simulink model "dspace"  (R2021b)
settings: Solver=FixedStepDiscrete  StartTime=0.0  StopTime=Inf  FixedStep=1e-3  RelTol=1e-3
PostLoadFcn:
  | , if any(exist('dsrtsu_mdlpostloadfcn', 'file') ~= 0), dsrtsu_mdlpostloadfcn('Execute', bdroot); end,
undefined symbols (not defined in the file): ami, amk1_setpoints_1, amk2_setpoints_1, amk3_setpoints_1, amk4_setpoints_1, as, digital, ebs, indicator, mcu_set_dbu_indicator_points, mcu_set_ecu_indicator_points, res_ntm_node_control
libraries: rtican x63, rti1401lib_dio_type3 x4, simulink x4, simulink_extras x1
(part 2 of 16)

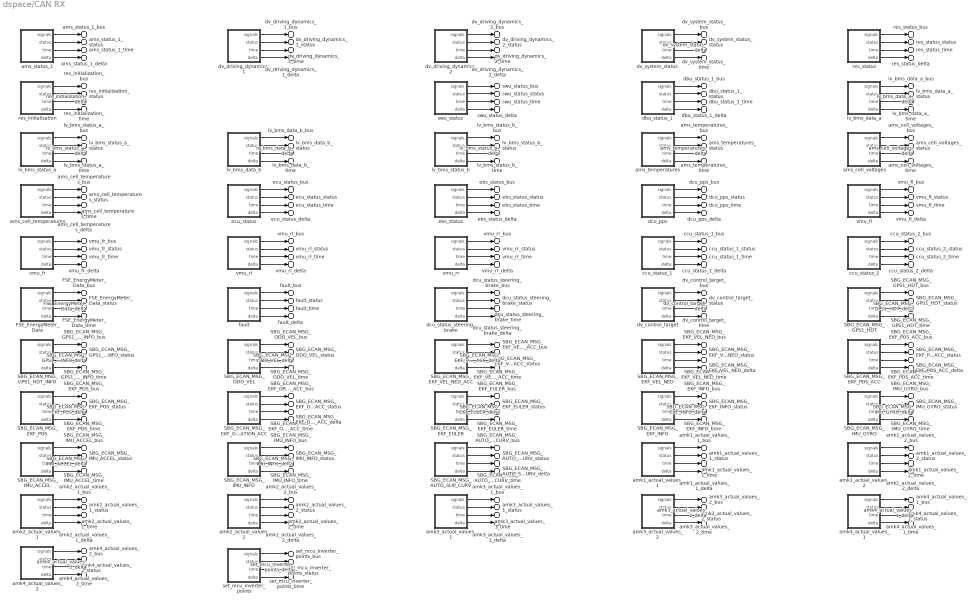
== system dspace/CAN RX ==
  FSE_EnergyMeter_Data : Subsystem
  SBG_ECAN_MSG_AUTO_SLIP_CURV : Subsystem
  SBG_ECAN_MSG_EKF_EULER : Subsystem
  SBG_ECAN_MSG_EKF_INFO : Subsystem
  SBG_ECAN_MSG_EKF_ORIENTATION_ACC : Subsystem
  SBG_ECAN_MSG_EKF_POS : Subsystem
  SBG_ECAN_MSG_EKF_POS_ACC : Subsystem
  SBG_ECAN_MSG_EKF_VEL_NED : Subsystem
  SBG_ECAN_MSG_EKF_VEL_NED_ACC : Subsystem
  SBG_ECAN_MSG_GPS1_HDT : Subsystem
  SBG_ECAN_MSG_GPS1_HDT_INFO : Subsystem
  SBG_ECAN_MSG_IMU_ACCEL : Subsystem
  SBG_ECAN_MSG_IMU_GYRO : Subsystem
  SBG_ECAN_MSG_IMU_INFO : Subsystem
  SBG_ECAN_MSG_ODO_VEL : Subsystem
  amk1_actual_values_1 : Subsystem
  amk1_actual_values_2 : Subsystem
  amk2_actual_values_1 : Subsystem
  amk2_actual_values_2 : Subsystem
  amk3_actual_values_1 : Subsystem
  amk3_actual_values_2 : Subsystem
  amk4_actual_values_1 : Subsystem
  amk4_actual_values_2 : Subsystem
  ams_cell_temperatures : Subsystem
  ams_cell_voltages : Subsystem
  ams_status_1 : Subsystem
  ams_temperatures : Subsystem
  ccu_status_1 : Subsystem
  ccu_status_2 : Subsystem
  dbu_status_1 : Subsystem
  dcu_pps : Subsystem
  dcu_status_steering_brake : Subsystem
  dv_control_target : Subsystem
  dv_driving_dynamics_1 : Subsystem
  dv_driving_dynamics_2 : Subsystem
  dv_system_status : Subsystem
  ebs_status : Subsystem
  ecu_status : Subsystem
  fault : Subsystem
  lv_bms_data_a : Subsystem
  lv_bms_data_b : Subsystem
  lv_bms_status_a : Subsystem
  lv_bms_status_b : Subsystem
  res_initialization : Subsystem
  res_status : Subsystem
  set_mcu_inverter_points : Subsystem
  swu_status : Subsystem
  vmu_fl : Subsystem
  vmu_fr : Subsystem
  vmu_rl : Subsystem
  vmu_rr : Subsystem
  lv_bms_status_a_bus : Outport  PortName=signals  Element=lv_bms_status_a
  lv_bms_data_b_bus : Outport  PortName=signals  Element=lv_bms_data_b
  lv_bms_status_b_bus : Outport  PortName=signals  Element=lv_bms_status_b
  ams_temperatures_bus : Outport  PortName=signals  Element=ams_temperatures
  ams_cell_voltages_bus : Outport  PortName=signals  Element=ams_cell_voltages
  ams_cell_temperatures_bus : Outport  PortName=signals  Element=ams_cell_temperatures
  ecu_status_bus : Outport  PortName=signals  Element=ecu_status
  ebs_status_bus : Outport  PortName=signals  Element=ebs_status
  dcu_pps_bus : Outport  PortName=signals  Element=dcu_pps
  vmu_fl_bus : Outport  PortName=signals  Element=vmu_fl
  vmu_fr_bus : Outport  PortName=signals  Element=vmu_fr
  vmu_rl_bus : Outport  PortName=signals  Element=vmu_rl
  vmu_rr_bus : Outport  PortName=signals  Element=vmu_rr
  ccu_status_1_bus : Outport  PortName=signals  Element=ccu_status_1
  ccu_status_2_bus : Outport  PortName=signals  Element=ccu_status_2
  FSE_EnergyMeter_Data_bus : Outport  PortName=signals  Element=FSE_EnergyMeter_Data
  fault_bus : Outport  PortName=signals  Element=fault
  dcu_status_steering_brake_bus : Outport  PortName=signals  Element=dcu_status_steering_brake
  dv_control_target_bus : Outport  PortName=signals  Element=dv_control_target
  SBG_ECAN_MSG_GPS1_HDT_bus : Outport  PortName=signals  Element=SBG_ECAN_MSG_GPS1_HDT
  SBG_ECAN_MSG_GPS1_HDT_INFO_bus : Outport  PortName=signals  Element=SBG_ECAN_MSG_GPS1_HDT_INFO
  SBG_ECAN_MSG_ODO_VEL_bus : Outport  PortName=signals  Element=SBG_ECAN_MSG_ODO_VEL
  SBG_ECAN_MSG_EKF_VEL_NED_ACC_bus : Outport  PortName=signals  Element=SBG_ECAN_MSG_EKF_VEL_NED_ACC
  SBG_ECAN_MSG_EKF_VEL_NED_bus : Outport  PortName=signals  Element=SBG_ECAN_MSG_EKF_VEL_NED
  SBG_ECAN_MSG_EKF_POS_ACC_bus : Outport  PortName=signals  Element=SBG_ECAN_MSG_EKF_POS_ACC
  SBG_ECAN_MSG_EKF_POS_bus : Outport  PortName=signals  Element=SBG_ECAN_MSG_EKF_POS
  SBG_ECAN_MSG_EKF_ORIENTATION_ACC_bus : Outport  PortName=signals  Element=SBG_ECAN_MSG_EKF_ORIENTATION_ACC
  SBG_ECAN_MSG_EKF_EULER_bus : Outport  PortName=signals  Element=SBG_ECAN_MSG_EKF_EULER
  SBG_ECAN_MSG_EKF_INFO_bus : Outport  PortName=signals  Element=SBG_ECAN_MSG_EKF_INFO
  SBG_ECAN_MSG_IMU_GYRO_bus : Outport  PortName=signals  Element=SBG_ECAN_MSG_IMU_GYRO
  SBG_ECAN_MSG_IMU_ACCEL_bus : Outport  PortName=signals  Element=SBG_ECAN_MSG_IMU_ACCEL
  SBG_ECAN_MSG_IMU_INFO_bus : Outport  PortName=signals  Element=SBG_ECAN_MSG_IMU_INFO
  SBG_ECAN_MSG_AUTO_SLIP_CURV_bus : Outport  PortName=signals  Element=SBG_ECAN_MSG_AUTO_SLIP_CURV
  amk1_actual_values_1_bus : Outport  PortName=signals  Element=amk1_actual_values_1
  amk1_actual_values_2_bus : Outport  PortName=signals  Element=amk1_actual_values_2
  amk2_actual_values_1_bus : Outport  PortName=signals  Element=amk2_actual_values_1
  amk2_actual_values_2_bus : Outport  PortName=signals  Element=amk2_actual_values_2
  amk3_actual_values_1_bus : Outport  PortName=signals  Element=amk3_actual_values_1
  amk3_actual_values_2_bus : Outport  PortName=signals  Element=amk3_actual_values_2
  amk4_actual_values_1_bus : Outport  PortName=signals  Element=amk4_actual_values_1
  amk4_actual_values_2_bus : Outport  PortName=signals  Element=amk4_actual_values_2
  ams_status_1_bus : Outport  PortName=signals  Element=ams_status_1
  dv_driving_dynamics_1_bus : Outport  PortName=signals  Element=dv_driving_dynamics_1
  dv_driving_dynamics_2_bus : Outport  PortName=signals  Element=dv_driving_dynamics_2
  dv_system_status_bus : Outport  PortName=signals  Element=dv_system_status
  res_status_bus : Outport  PortName=signals  Element=res_status
  res_initialization_bus : Outport  PortName=signals  Element=res_initialization
  swu_status_bus : Outport  PortName=signals  Element=swu_status
  dbu_status_1_bus : Outport  PortName=signals  Element=dbu_status_1
  lv_bms_data_a_bus : Outport  PortName=signals  Element=lv_bms_data_a
  set_mcu_inverter_points_bus : Outport  PortName=signals  Element=set_mcu_inverter_points
  lv_bms_status_a_delta : Outport  Port=2  PortName=deltas  Element=lv_bms_status_a_delta
  lv_bms_data_b_delta : Outport  Port=2  PortName=deltas  Element=lv_bms_data_b_delta
  lv_bms_status_b_delta : Outport  Port=2  PortName=deltas  Element=lv_bms_status_b_delta
  ams_temperatures_delta : Outport  Port=2  PortName=deltas  Element=ams_temperatures_delta
  ams_cell_voltages_delta : Outport  Port=2  PortName=deltas  Element=ams_cell_voltages_delta
  ams_cell_temperatures_delta : Outport  Port=2  PortName=deltas  Element=ams_cell_temperatures_delta
  ecu_status_delta : Outport  Port=2  PortName=deltas  Element=ecu_status_delta
  ebs_status_delta : Outport  Port=2  PortName=deltas  Element=ebs_status_delta
  dcu_pps_delta : Outport  Port=2  PortName=deltas  Element=dcu_pps_delta
  vmu_fl_delta : Outport  Port=2  PortName=deltas  Element=vmu_fl_delta
  vmu_fr_delta : Outport  Port=2  PortName=deltas  Element=vmu_fr_delta
  vmu_rl_delta : Outport  Port=2  PortName=deltas  Element=vmu_rl_delta
  vmu_rr_delta : Outport  Port=2  PortName=deltas  Element=vmu_rr_delta
  ccu_status_1_delta : Outport  Port=2  PortName=deltas  Element=ccu_status_1_delta
  ccu_status_2_delta : Outport  Port=2  PortName=deltas  Element=ccu_status_2_delta
  FSE_EnergyMeter_Data_delta : Outport  Port=2  PortName=deltas  Element=FSE_EnergyMeter_Data_delta
  fault_delta : Outport  Port=2  PortName=deltas  Element=fault_delta
  dcu_status_steering_brake_delta : Outport  Port=2  PortName=deltas  Element=dcu_status_steering_brake_delta
  dv_control_target_delta : Outport  Port=2  PortName=deltas  Element=dv_control_target_delta
  SBG_ECAN_MSG_GPS1_HDT_delta : Outport  Port=2  PortName=deltas  Element=SBG_ECAN_MSG_GPS1_HDT_delta
  SBG_ECAN_MSG_GPS1_HDT_INFO_delta : Outport  Port=2  PortName=deltas  Element=SBG_ECAN_MSG_GPS1_HDT_INFO_delta
  SBG_ECAN_MSG_ODO_VEL_delta : Outport  Port=2  PortName=deltas  Element=SBG_ECAN_MSG_ODO_VEL_delta
  SBG_ECAN_MSG_EKF_VEL_NED_ACC_delta : Outport  Port=2  PortName=deltas  Element=SBG_ECAN_MSG_EKF_VEL_NED_ACC_delta
  SBG_ECAN_MSG_EKF_VEL_NED_delta : Outport  Port=2  PortName=deltas  Element=SBG_ECAN_MSG_EKF_VEL_NED_delta
  SBG_ECAN_MSG_EKF_POS_ACC_delta : Outport  Port=2  PortName=deltas  Element=SBG_ECAN_MSG_EKF_POS_ACC_delta
  SBG_ECAN_MSG_EKF_POS_delta : Outport  Port=2  PortName=deltas  Element=SBG_ECAN_MSG_EKF_POS_delta
  SBG_ECAN_MSG_EKF_ORIENTATION_ACC_delta : Outport  Port=2  PortName=deltas  Element=SBG_ECAN_MSG_EKF_ORIENTATION_ACC_delta
  SBG_ECAN_MSG_EKF_EULER_delta : Outport  Port=2  PortName=deltas  Element=SBG_ECAN_MSG_EKF_EULER_delta
  SBG_ECAN_MSG_EKF_INFO_delta : Outport  Port=2  PortName=deltas  Element=SBG_ECAN_MSG_EKF_INFO_delta
  SBG_ECAN_MSG_IMU_GYRO_delta : Outport  Port=2  PortName=deltas  Element=SBG_ECAN_MSG_IMU_GYRO_delta
  SBG_ECAN_MSG_IMU_ACCEL_delta : Outport  Port=2  PortName=deltas  Element=SBG_ECAN_MSG_IMU_ACCEL_delta
  SBG_ECAN_MSG_IMU_INFO_delta : Outport  Port=2  PortName=deltas  Element=SBG_ECAN_MSG_IMU_INFO_delta
  SBG_ECAN_MSG_AUTO_SLIP_CURV_delta : Outport  Port=2  PortName=deltas  Element=SBG_ECAN_MSG_AUTO_SLIP_CURV_delta
  amk1_actual_values_1_delta : Outport  Port=2  PortName=deltas  Element=amk1_actual_values_1_delta
  amk1_actual_values_2_delta : Outport  Port=2  PortName=deltas  Element=amk1_actual_values_2_delta
  amk2_actual_values_1_delta : Outport  Port=2  PortName=deltas  Element=amk2_actual_values_1_delta
  amk2_actual_values_2_delta : Outport  Port=2  PortName=deltas  Element=amk2_actual_values_2_delta
  amk3_actual_values_1_delta : Outport  Port=2  PortName=deltas  Element=amk3_actual_values_1_delta
  amk3_actual_values_2_delta : Outport  Port=2  PortName=deltas  Element=amk3_actual_values_2_delta
  amk4_actual_values_1_delta : Outport  Port=2  PortName=deltas  Element=amk4_actual_values_1_delta
  amk4_actual_values_2_delta : Outport  Port=2  PortName=deltas  Element=amk4_actual_values_2_delta
  ams_status_1_delta : Outport  Port=2  PortName=deltas  Element=ams_status_1_delta
  dv_driving_dynamics_1_delta : Outport  Port=2  PortName=deltas  Element=dv_driving_dynamics_1_delta
  dv_driving_dynamics_2_delta : Outport  Port=2  PortName=deltas  Element=dv_driving_dynamics_2_delta
  dv_system_status_delta : Outport  Port=2  PortName=deltas  Element=dv_system_status_delta
  res_status_delta : Outport  Port=2  PortName=deltas  Element=res_status_delta
  res_initialization_delta : Outport  Port=2  PortName=deltas  Element=res_initialization_delta
  swu_status_delta : Outport  Port=2  PortName=deltas  Element=swu_status_delta
  dbu_status_1_delta : Outport  Port=2  PortName=deltas  Element=dbu_status_1_delta
  lv_bms_data_a_delta : Outport  Port=2  PortName=deltas  Element=lv_bms_data_a_delta
  set_mcu_inverter_points_delta : Outport  Port=2  PortName=deltas  Element=set_mcu_inverter_points_delta
  lv_bms_status_a_status : Outport  Port=3  PortName=status  Element=lv_bms_status_a_status
  lv_bms_data_b_status : Outport  Port=3  PortName=status  Element=lv_bms_data_b_status
  lv_bms_status_b_status : Outport  Port=3  PortName=status  Element=lv_bms_status_b_status
  ams_temperatures_status : Outport  Port=3  PortName=status  Element=ams_temperatures_status
  ams_cell_voltages_status : Outport  Port=3  PortName=status  Element=ams_cell_voltages_status
  ams_cell_temperatures_status : Outport  Port=3  PortName=status  Element=ams_cell_temperatures_status
  ecu_status_status : Outport  Port=3  PortName=status  Element=ecu_status_status
  ebs_status_status : Outport  Port=3  PortName=status  Element=ebs_status_status
  dcu_pps_status : Outport  Port=3  PortName=status  Element=dcu_pps_status
  vmu_fl_status : Outport  Port=3  PortName=status  Element=vmu_fl_status
  vmu_fr_status : Outport  Port=3  PortName=status  Element=vmu_fr_status
  vmu_rl_status : Outport  Port=3  PortName=status  Element=vmu_rl_status
  vmu_rr_status : Outport  Port=3  PortName=status  Element=vmu_rr_status
  ccu_status_1_status : Outport  Port=3  PortName=status  Element=ccu_status_1_status
  ccu_status_2_status : Outport  Port=3  PortName=status  Element=ccu_status_2_status
  FSE_EnergyMeter_Data_status : Outport  Port=3  PortName=status  Element=FSE_EnergyMeter_Data_status
  fault_status : Outport  Port=3  PortName=status  Element=fault_status
  dcu_status_steering_brake_status : Outport  Port=3  PortName=status  Element=dcu_status_steering_brake_status
  dv_control_target_status : Outport  Port=3  PortName=status  Element=dv_control_target_status
  SBG_ECAN_MSG_GPS1_HDT_status : Outport  Port=3  PortName=status  Element=SBG_ECAN_MSG_GPS1_HDT_status
  SBG_ECAN_MSG_GPS1_HDT_INFO_status : Outport  Port=3  PortName=status  Element=SBG_ECAN_MSG_GPS1_HDT_INFO_status
  SBG_ECAN_MSG_ODO_VEL_status : Outport  Port=3  PortName=status  Element=SBG_ECAN_MSG_ODO_VEL_status
  SBG_ECAN_MSG_EKF_VEL_NED_ACC_status : Outport  Port=3  PortName=status  Element=SBG_ECAN_MSG_EKF_VEL_NED_ACC_status
  SBG_ECAN_MSG_EKF_VEL_NED_status : Outport  Port=3  PortName=status  Element=SBG_ECAN_MSG_EKF_VEL_NED_status
  SBG_ECAN_MSG_EKF_POS_ACC_status : Outport  Port=3  PortName=status  Element=SBG_ECAN_MSG_EKF_POS_ACC_status
  SBG_ECAN_MSG_EKF_POS_status : Outport  Port=3  PortName=status  Element=SBG_ECAN_MSG_EKF_POS_status
  SBG_ECAN_MSG_EKF_ORIENTATION_ACC_status : Outport  Port=3  PortName=status  Element=SBG_ECAN_MSG_EKF_ORIENTATION_ACC_status
  SBG_ECAN_MSG_EKF_EULER_status : Outport  Port=3  PortName=status  Element=SBG_ECAN_MSG_EKF_EULER_status
  SBG_ECAN_MSG_EKF_INFO_status : Outport  Port=3  PortName=status  Element=SBG_ECAN_MSG_EKF_INFO_status
  SBG_ECAN_MSG_IMU_GYRO_status : Outport  Port=3  PortName=status  Element=SBG_ECAN_MSG_IMU_GYRO_status
  SBG_ECAN_MSG_IMU_ACCEL_status : Outport  Port=3  PortName=status  Element=SBG_ECAN_MSG_IMU_ACCEL_status
  SBG_ECAN_MSG_IMU_INFO_status : Outport  Port=3  PortName=status  Element=SBG_ECAN_MSG_IMU_INFO_status
  SBG_ECAN_MSG_AUTO_SLIP_CURV_status : Outport  Port=3  PortName=status  Element=SBG_ECAN_MSG_AUTO_SLIP_CURV_status
  amk1_actual_values_1_status : Outport  Port=3  PortName=status  Element=amk1_actual_values_1_status
  amk1_actual_values_2_status : Outport  Port=3  PortName=status  Element=amk1_actual_values_2_status
  amk2_actual_values_1_status : Outport  Port=3  PortName=status  Element=amk2_actual_values_1_status
  amk2_actual_values_2_status : Outport  Port=3  PortName=status  Element=amk2_actual_values_2_status
  amk3_actual_values_1_status : Outport  Port=3  PortName=status  Element=amk3_actual_values_1_status
  amk3_actual_values_2_status : Outport  Port=3  PortName=status  Element=amk3_actual_values_2_status
  amk4_actual_values_1_status : Outport  Port=3  PortName=status  Element=amk4_actual_values_1_status
  amk4_actual_values_2_status : Outport  Port=3  PortName=status  Element=amk4_actual_values_2_status
  ams_status_1_status : Outport  Port=3  PortName=status  Element=ams_status_1_status
  dv_driving_dynamics_1_status : Outport  Port=3  PortName=status  Element=dv_driving_dynamics_1_status
  dv_driving_dynamics_2_status : Outport  Port=3  PortName=status  Element=dv_driving_dynamics_2_status
  dv_system_status_status : Outport  Port=3  PortName=status  Element=dv_system_status_status
  res_status_status : Outport  Port=3  PortName=status  Element=res_status_status
  res_initialization_status : Outport  Port=3  PortName=status  Element=res_initialization_status
  swu_status_status : Outport  Port=3  PortName=status  Element=swu_status_status
  dbu_status_1_status : Outport  Port=3  PortName=status  Element=dbu_status_1_status
  lv_bms_data_a_status : Outport  Port=3  PortName=status  Element=lv_bms_data_a_status
  set_mcu_inverter_points_status : Outport  Port=3  PortName=status  Element=set_mcu_inverter_points_status
  lv_bms_status_a_time : Outport  Port=4  PortName=time  Element=lv_bms_status_a_time
  lv_bms_data_b_time : Outport  Port=4  PortName=time  Element=lv_bms_data_b_time
  lv_bms_status_b_time : Outport  Port=4  PortName=time  Element=lv_bms_status_b_time
  ams_temperatures_time : Outport  Port=4  PortName=time  Element=ams_temperatures_time
  ams_cell_voltages_time : Outport  Port=4  PortName=time  Element=ams_cell_voltages_time
  ams_cell_temperatures_time : Outport  Port=4  PortName=time  Element=ams_cell_temperatures_time
  ecu_status_time : Outport  Port=4  PortName=time  Element=ecu_status_time
  ebs_status_time : Outport  Port=4  PortName=time  Element=ebs_status_time
  dcu_pps_time : Outport  Port=4  PortName=time  Element=dcu_pps_time
  vmu_fl_time : Outport  Port=4  PortName=time  Element=vmu_fl_time
  vmu_fr_time : Outport  Port=4  PortName=time  Element=vmu_fr_time
  vmu_rl_time : Outport  Port=4  PortName=time  Element=vmu_rl_time
  vmu_rr_time : Outport  Port=4  PortName=time  Element=vmu_rr_time
  ccu_status_1_time : Outport  Port=4  PortName=time  Element=ccu_status_1_time
  ccu_status_2_time : Outport  Port=4  PortName=time  Element=ccu_status_2_time
  FSE_EnergyMeter_Data_time : Outport  Port=4  PortName=time  Element=FSE_EnergyMeter_Data_time
  fault_time : Outport  Port=4  PortName=time  Element=fault_time
  dcu_status_steering_brake_time : Outport  Port=4  PortName=time  Element=dcu_status_steering_brake_time
  dv_control_target_time : Outport  Port=4  PortName=time  Element=dv_control_target_time
  SBG_ECAN_MSG_GPS1_HDT_time : Outport  Port=4  PortName=time  Element=SBG_ECAN_MSG_GPS1_HDT_time
  SBG_ECAN_MSG_GPS1_HDT_INFO_time : Outport  Port=4  PortName=time  Element=SBG_ECAN_MSG_GPS1_HDT_INFO_time
  SBG_ECAN_MSG_ODO_VEL_time : Outport  Port=4  PortName=time  Element=SBG_ECAN_MSG_ODO_VEL_time
  SBG_ECAN_MSG_EKF_VEL_NED_ACC_time : Outport  Port=4  PortName=time  Element=SBG_ECAN_MSG_EKF_VEL_NED_ACC_time
  SBG_ECAN_MSG_EKF_VEL_NED_time : Outport  Port=4  PortName=time  Element=SBG_ECAN_MSG_EKF_VEL_NED_time
  SBG_ECAN_MSG_EKF_POS_ACC_time : Outport  Port=4  PortName=time  Element=SBG_ECAN_MSG_EKF_POS_ACC_time
  SBG_ECAN_MSG_EKF_POS_time : Outport  Port=4  PortName=time  Element=SBG_ECAN_MSG_EKF_POS_time
  SBG_ECAN_MSG_EKF_ORIENTATION_ACC_time : Outport  Port=4  PortName=time  Element=SBG_ECAN_MSG_EKF_ORIENTATION_ACC_time
  SBG_ECAN_MSG_EKF_EULER_time : Outport  Port=4  PortName=time  Element=SBG_ECAN_MSG_EKF_EULER_time
  SBG_ECAN_MSG_EKF_INFO_time : Outport  Port=4  PortName=time  Element=SBG_ECAN_MSG_EKF_INFO_time
  SBG_ECAN_MSG_IMU_GYRO_time : Outport  Port=4  PortName=time  Element=SBG_ECAN_MSG_IMU_GYRO_time
  SBG_ECAN_MSG_IMU_ACCEL_time : Outport  Port=4  PortName=time  Element=SBG_ECAN_MSG_IMU_ACCEL_time
  SBG_ECAN_MSG_IMU_INFO_time : Outport  Port=4  PortName=time  Element=SBG_ECAN_MSG_IMU_INFO_time
  SBG_ECAN_MSG_AUTO_SLIP_CURV_time : Outport  Port=4  PortName=time  Element=SBG_ECAN_MSG_AUTO_SLIP_CURV_time
  amk1_actual_values_1_time : Outport  Port=4  PortName=time  Element=amk1_actual_values_1_time
  amk1_actual_values_2_time : Outport  Port=4  PortName=time  Element=amk1_actual_values_2_time
  amk2_actual_values_1_time : Outport  Port=4  PortName=time  Element=amk2_actual_values_1_time
  amk2_actual_values_2_time : Outport  Port=4  PortName=time  Element=amk2_actual_values_2_time
  amk3_actual_values_1_time : Outport  Port=4  PortName=time  Element=amk3_actual_values_1_time
  amk3_actual_values_2_time : Outport  Port=4  PortName=time  Element=amk3_actual_values_2_time
  amk4_actual_values_1_time : Outport  Port=4  PortName=time  Element=amk4_actual_values_1_time
  amk4_actual_values_2_time : Outport  Port=4  PortName=time  Element=amk4_actual_values_2_time
  ams_status_1_time : Outport  Port=4  PortName=time  Element=ams_status_1_time
  dv_driving_dynamics_1_time : Outport  Port=4  PortName=time  Element=dv_driving_dynamics_1_time
  dv_driving_dynamics_2_time : Outport  Port=4  PortName=time  Element=dv_driving_dynamics_2_time
  dv_system_status_time : Outport  Port=4  PortName=time  Element=dv_system_status_time
  res_status_time : Outport  Port=4  PortName=time  Element=res_status_time
  res_initialization_time : Outport  Port=4  PortName=time  Element=res_initialization_time
  swu_status_time : Outport  Port=4  PortName=time  Element=swu_status_time
  dbu_status_1_time : Outport  Port=4  PortName=time  Element=dbu_status_1_time
  lv_bms_data_a_time : Outport  Port=4  PortName=time  Element=lv_bms_data_a_time
  set_mcu_inverter_points_time : Outport  Port=4  PortName=time  Element=set_mcu_inverter_points_time
  wires:
  lv_bms_status_a/1(signals) -> lv_bms_status_a_bus/1
  lv_bms_status_a/2(status) -> lv_bms_status_a_status/1
  lv_bms_status_a/3(time) -> lv_bms_status_a_time/1
  lv_bms_status_a/4(delta) -> lv_bms_status_a_delta/1
  lv_bms_data_b/1(signals) -> lv_bms_data_b_bus/1
  lv_bms_data_b/2(status) -> lv_bms_data_b_status/1
  lv_bms_data_b/3(time) -> lv_bms_data_b_time/1
  lv_bms_data_b/4(delta) -> lv_bms_data_b_delta/1
  lv_bms_status_b/1(signals) -> lv_bms_status_b_bus/1
  lv_bms_status_b/2(status) -> lv_bms_status_b_status/1
  lv_bms_status_b/3(time) -> lv_bms_status_b_time/1
  lv_bms_status_b/4(delta) -> lv_bms_status_b_delta/1
  ams_temperatures/1(signals) -> ams_temperatures_bus/1
  ams_temperatures/2(status) -> ams_temperatures_status/1
  ams_temperatures/3(time) -> ams_temperatures_time/1
  ams_temperatures/4(delta) -> ams_temperatures_delta/1
  ams_cell_voltages/1(signals) -> ams_cell_voltages_bus/1
  ams_cell_voltages/2(status) -> ams_cell_voltages_status/1
  ams_cell_voltages/3(time) -> ams_cell_voltages_time/1
  ams_cell_voltages/4(delta) -> ams_cell_voltages_delta/1
  ams_cell_temperatures/1(signals) -> ams_cell_temperatures_bus/1
  ams_cell_temperatures/2(status) -> ams_cell_temperatures_status/1
  ams_cell_temperatures/3(time) -> ams_cell_temperatures_time/1
  ams_cell_temperatures/4(delta) -> ams_cell_temperatures_delta/1
  ecu_status/1(signals) -> ecu_status_bus/1
  ecu_status/2(status) -> ecu_status_status/1
  ecu_status/3(time) -> ecu_status_time/1
  ecu_status/4(delta) -> ecu_status_delta/1
  ebs_status/1(signals) -> ebs_status_bus/1
  ebs_status/2(status) -> ebs_status_status/1
  ebs_status/3(time) -> ebs_status_time/1
  ebs_status/4(delta) -> ebs_status_delta/1
  dcu_pps/1(signals) -> dcu_pps_bus/1
  dcu_pps/2(status) -> dcu_pps_status/1
  dcu_pps/3(time) -> dcu_pps_time/1
  dcu_pps/4(delta) -> dcu_pps_delta/1
  vmu_fl/1(signals) -> vmu_fl_bus/1
  vmu_fl/2(status) -> vmu_fl_status/1
  vmu_fl/3(time) -> vmu_fl_time/1
  vmu_fl/4(delta) -> vmu_fl_delta/1
  vmu_fr/1(signals) -> vmu_fr_bus/1
  vmu_fr/2(status) -> vmu_fr_status/1
  vmu_fr/3(time) -> vmu_fr_time/1
  vmu_fr/4(delta) -> vmu_fr_delta/1
  vmu_rl/1(signals) -> vmu_rl_bus/1
  vmu_rl/2(status) -> vmu_rl_status/1
  vmu_rl/3(time) -> vmu_rl_time/1
  vmu_rl/4(delta) -> vmu_rl_delta/1
  vmu_rr/1(signals) -> vmu_rr_bus/1
  vmu_rr/2(status) -> vmu_rr_status/1
  vmu_rr/3(time) -> vmu_rr_time/1
  vmu_rr/4(delta) -> vmu_rr_delta/1
  ccu_status_1/1(signals) -> ccu_status_1_bus/1
  ccu_status_1/2(status) -> ccu_status_1_status/1
  ccu_status_1/3(time) -> ccu_status_1_time/1
  ccu_status_1/4(delta) -> ccu_status_1_delta/1
  ccu_status_2/1(signals) -> ccu_status_2_bus/1
  ccu_status_2/2(status) -> ccu_status_2_status/1
  ccu_status_2/3(time) -> ccu_status_2_time/1
  ccu_status_2/4(delta) -> ccu_status_2_delta/1
  FSE_EnergyMeter_Data/1(signals) -> FSE_EnergyMeter_Data_bus/1
  FSE_EnergyMeter_Data/2(status) -> FSE_EnergyMeter_Data_status/1
  FSE_EnergyMeter_Data/3(time) -> FSE_EnergyMeter_Data_time/1
  FSE_EnergyMeter_Data/4(delta) -> FSE_EnergyMeter_Data_delta/1
  fault/1(signals) -> fault_bus/1
  fault/2(status) -> fault_status/1
  fault/3(time) -> fault_time/1
  fault/4(delta) -> fault_delta/1
  dcu_status_steering_brake/1(signals) -> dcu_status_steering_brake_bus/1
  dcu_status_steering_brake/2(status) -> dcu_status_steering_brake_status/1
  dcu_status_steering_brake/3(time) -> dcu_status_steering_brake_time/1
  dcu_status_steering_brake/4(delta) -> dcu_status_steering_brake_delta/1
  dv_control_target/1(signals) -> dv_control_target_bus/1
  dv_control_target/2(status) -> dv_control_target_status/1
  dv_control_target/3(time) -> dv_control_target_time/1
  dv_control_target/4(delta) -> dv_control_target_delta/1
  SBG_ECAN_MSG_GPS1_HDT/1(signals) -> SBG_ECAN_MSG_GPS1_HDT_bus/1
  SBG_ECAN_MSG_GPS1_HDT/2(status) -> SBG_ECAN_MSG_GPS1_HDT_status/1
  SBG_ECAN_MSG_GPS1_HDT/3(time) -> SBG_ECAN_MSG_GPS1_HDT_time/1
  SBG_ECAN_MSG_GPS1_HDT/4(delta) -> SBG_ECAN_MSG_GPS1_HDT_delta/1
  SBG_ECAN_MSG_GPS1_HDT_INFO/1(signals) -> SBG_ECAN_MSG_GPS1_HDT_INFO_bus/1
  SBG_ECAN_MSG_GPS1_HDT_INFO/2(status) -> SBG_ECAN_MSG_GPS1_HDT_INFO_status/1
  SBG_ECAN_MSG_GPS1_HDT_INFO/3(time) -> SBG_ECAN_MSG_GPS1_HDT_INFO_time/1
  SBG_ECAN_MSG_GPS1_HDT_INFO/4(delta) -> SBG_ECAN_MSG_GPS1_HDT_INFO_delta/1
  SBG_ECAN_MSG_ODO_VEL/1(signals) -> SBG_ECAN_MSG_ODO_VEL_bus/1
  SBG_ECAN_MSG_ODO_VEL/2(status) -> SBG_ECAN_MSG_ODO_VEL_status/1
  SBG_ECAN_MSG_ODO_VEL/3(time) -> SBG_ECAN_MSG_ODO_VEL_time/1
  SBG_ECAN_MSG_ODO_VEL/4(delta) -> SBG_ECAN_MSG_ODO_VEL_delta/1
  SBG_ECAN_MSG_EKF_VEL_NED_ACC/1(signals) -> SBG_ECAN_MSG_EKF_VEL_NED_ACC_bus/1
  SBG_ECAN_MSG_EKF_VEL_NED_ACC/2(status) -> SBG_ECAN_MSG_EKF_VEL_NED_ACC_status/1
  SBG_ECAN_MSG_EKF_VEL_NED_ACC/3(time) -> SBG_ECAN_MSG_EKF_VEL_NED_ACC_time/1
  SBG_ECAN_MSG_EKF_VEL_NED_ACC/4(delta) -> SBG_ECAN_MSG_EKF_VEL_NED_ACC_delta/1
  SBG_ECAN_MSG_EKF_VEL_NED/1(signals) -> SBG_ECAN_MSG_EKF_VEL_NED_bus/1
  SBG_ECAN_MSG_EKF_VEL_NED/2(status) -> SBG_ECAN_MSG_EKF_VEL_NED_status/1
  SBG_ECAN_MSG_EKF_VEL_NED/3(time) -> SBG_ECAN_MSG_EKF_VEL_NED_time/1
  SBG_ECAN_MSG_EKF_VEL_NED/4(delta) -> SBG_ECAN_MSG_EKF_VEL_NED_delta/1
  SBG_ECAN_MSG_EKF_POS_ACC/1(signals) -> SBG_ECAN_MSG_EKF_POS_ACC_bus/1
  SBG_ECAN_MSG_EKF_POS_ACC/2(status) -> SBG_ECAN_MSG_EKF_POS_ACC_status/1
  SBG_ECAN_MSG_EKF_POS_ACC/3(time) -> SBG_ECAN_MSG_EKF_POS_ACC_time/1
  SBG_ECAN_MSG_EKF_POS_ACC/4(delta) -> SBG_ECAN_MSG_EKF_POS_ACC_delta/1
  SBG_ECAN_MSG_EKF_POS/1(signals) -> SBG_ECAN_MSG_EKF_POS_bus/1
  SBG_ECAN_MSG_EKF_POS/2(status) -> SBG_ECAN_MSG_EKF_POS_status/1
  SBG_ECAN_MSG_EKF_POS/3(time) -> SBG_ECAN_MSG_EKF_POS_time/1
  SBG_ECAN_MSG_EKF_POS/4(delta) -> SBG_ECAN_MSG_EKF_POS_delta/1
  SBG_ECAN_MSG_EKF_ORIENTATION_ACC/1(signals) -> SBG_ECAN_MSG_EKF_ORIENTATION_ACC_bus/1
  SBG_ECAN_MSG_EKF_ORIENTATION_ACC/2(status) -> SBG_ECAN_MSG_EKF_ORIENTATION_ACC_status/1
  SBG_ECAN_MSG_EKF_ORIENTATION_ACC/3(time) -> SBG_ECAN_MSG_EKF_ORIENTATION_ACC_time/1
  SBG_ECAN_MSG_EKF_ORIENTATION_ACC/4(delta) -> SBG_ECAN_MSG_EKF_ORIENTATION_ACC_delta/1
  SBG_ECAN_MSG_EKF_EULER/1(signals) -> SBG_ECAN_MSG_EKF_EULER_bus/1
  SBG_ECAN_MSG_EKF_EULER/2(status) -> SBG_ECAN_MSG_EKF_EULER_status/1
  SBG_ECAN_MSG_EKF_EULER/3(time) -> SBG_ECAN_MSG_EKF_EULER_time/1
  SBG_ECAN_MSG_EKF_EULER/4(delta) -> SBG_ECAN_MSG_EKF_EULER_delta/1
  SBG_ECAN_MSG_EKF_INFO/1(signals) -> SBG_ECAN_MSG_EKF_INFO_bus/1
  SBG_ECAN_MSG_EKF_INFO/2(status) -> SBG_ECAN_MSG_EKF_INFO_status/1
  SBG_ECAN_MSG_EKF_INFO/3(time) -> SBG_ECAN_MSG_EKF_INFO_time/1
  SBG_ECAN_MSG_EKF_INFO/4(delta) -> SBG_ECAN_MSG_EKF_INFO_delta/1
  SBG_ECAN_MSG_IMU_GYRO/1(signals) -> SBG_ECAN_MSG_IMU_GYRO_bus/1
  SBG_ECAN_MSG_IMU_GYRO/2(status) -> SBG_ECAN_MSG_IMU_GYRO_status/1
  SBG_ECAN_MSG_IMU_GYRO/3(time) -> SBG_ECAN_MSG_IMU_GYRO_time/1
  SBG_ECAN_MSG_IMU_GYRO/4(delta) -> SBG_ECAN_MSG_IMU_GYRO_delta/1
  SBG_ECAN_MSG_IMU_ACCEL/1(signals) -> SBG_ECAN_MSG_IMU_ACCEL_bus/1
  SBG_ECAN_MSG_IMU_ACCEL/2(status) -> SBG_ECAN_MSG_IMU_ACCEL_status/1
  SBG_ECAN_MSG_IMU_ACCEL/3(time) -> SBG_ECAN_MSG_IMU_ACCEL_time/1
  SBG_ECAN_MSG_IMU_ACCEL/4(delta) -> SBG_ECAN_MSG_IMU_ACCEL_delta/1
  SBG_ECAN_MSG_IMU_INFO/1(signals) -> SBG_ECAN_MSG_IMU_INFO_bus/1
  SBG_ECAN_MSG_IMU_INFO/2(status) -> SBG_ECAN_MSG_IMU_INFO_status/1
  SBG_ECAN_MSG_IMU_INFO/3(time) -> SBG_ECAN_MSG_IMU_INFO_time/1
  SBG_ECAN_MSG_IMU_INFO/4(delta) -> SBG_ECAN_MSG_IMU_INFO_delta/1
  SBG_ECAN_MSG_AUTO_SLIP_CURV/1(signals) -> SBG_ECAN_MSG_AUTO_SLIP_CURV_bus/1
  SBG_ECAN_MSG_AUTO_SLIP_CURV/2(status) -> SBG_ECAN_MSG_AUTO_SLIP_CURV_status/1
  SBG_ECAN_MSG_AUTO_SLIP_CURV/3(time) -> SBG_ECAN_MSG_AUTO_SLIP_CURV_time/1
  SBG_ECAN_MSG_AUTO_SLIP_CURV/4(delta) -> SBG_ECAN_MSG_AUTO_SLIP_CURV_delta/1
  amk1_actual_values_1/1(signals) -> amk1_actual_values_1_bus/1
  amk1_actual_values_1/2(status) -> amk1_actual_values_1_status/1
  amk1_actual_values_1/3(time) -> amk1_actual_values_1_time/1
  amk1_actual_values_1/4(delta) -> amk1_actual_values_1_delta/1
  amk1_actual_values_2/1(signals) -> amk1_actual_values_2_bus/1
  amk1_actual_values_2/2(status) -> amk1_actual_values_2_status/1
  amk1_actual_values_2/3(time) -> amk1_actual_values_2_time/1
  amk1_actual_values_2/4(delta) -> amk1_actual_values_2_delta/1
  amk2_actual_values_1/1(signals) -> amk2_actual_values_1_bus/1
  amk2_actual_values_1/2(status) -> amk2_actual_values_1_status/1
  amk2_actual_values_1/3(time) -> amk2_actual_values_1_time/1
  amk2_actual_values_1/4(delta) -> amk2_actual_values_1_delta/1
  amk2_actual_values_2/1(signals) -> amk2_actual_values_2_bus/1
  amk2_actual_values_2/2(status) -> amk2_actual_values_2_status/1
  amk2_actual_values_2/3(time) -> amk2_actual_values_2_time/1
  amk2_actual_values_2/4(delta) -> amk2_actual_values_2_delta/1
  amk3_actual_values_1/1(signals) -> amk3_actual_values_1_bus/1
  amk3_actual_values_1/2(status) -> amk3_actual_values_1_status/1
  amk3_actual_values_1/3(time) -> amk3_actual_values_1_time/1
  amk3_actual_values_1/4(delta) -> amk3_actual_values_1_delta/1
  amk3_actual_values_2/1(signals) -> amk3_actual_values_2_bus/1
  amk3_actual_values_2/2(status) -> amk3_actual_values_2_status/1
  amk3_actual_values_2/3(time) -> amk3_actual_values_2_time/1
  amk3_actual_values_2/4(delta) -> amk3_actual_values_2_delta/1
  amk4_actual_values_1/1(signals) -> amk4_actual_values_1_bus/1
  amk4_actual_values_1/2(status) -> amk4_actual_values_1_status/1
  amk4_actual_values_1/3(time) -> amk4_actual_values_1_time/1
  amk4_actual_values_1/4(delta) -> amk4_actual_values_1_delta/1
  amk4_actual_values_2/1(signals) -> amk4_actual_values_2_bus/1
  amk4_actual_values_2/2(status) -> amk4_actual_values_2_status/1
  amk4_actual_values_2/3(time) -> amk4_actual_values_2_time/1
  amk4_actual_values_2/4(delta) -> amk4_actual_values_2_delta/1
  swu_status/4(delta) -> swu_status_delta/1
  dv_system_status/3(time) -> dv_system_status_time/1
  ams_status_1/3(time) -> ams_status_1_time/1
  dv_driving_dynamics_2/2(status) -> dv_driving_dynamics_2_status/1
  dv_system_status/1(signals) -> dv_system_status_bus/1
  dbu_status_1/1(signals) -> dbu_status_1_bus/1
  dv_driving_dynamics_1/3(time) -> dv_driving_dynamics_1_time/1
  res_initialization/3(time) -> res_initialization_time/1
  dbu_status_1/2(status) -> dbu_status_1_status/1
  res_status/1(signals) -> res_status_bus/1
  swu_status/2(status) -> swu_status_status/1
  lv_bms_data_a/4(delta) -> lv_bms_data_a_delta/1
  res_initialization/4(delta) -> res_initialization_delta/1
  swu_status/3(time) -> swu_status_time/1
  swu_status/1(signals) -> swu_status_bus/1
  res_status/3(time) -> res_status_time/1
  ams_status_1/1(signals) -> ams_status_1_bus/1
  dbu_status_1/3(time) -> dbu_status_1_time/1
  res_status/4(delta) -> res_status_delta/1
  res_initialization/1(signals) -> res_initialization_bus/1
  lv_bms_data_a/3(time) -> lv_bms_data_a_time/1
  dv_driving_dynamics_1/1(signals) -> dv_driving_dynamics_1_bus/1
  res_status/2(status) -> res_status_status/1
  dv_system_status/4(delta) -> dv_system_status_delta/1
  dv_system_status/2(status) -> dv_system_status_status/1
  ams_status_1/2(status) -> ams_status_1_status/1
  dv_driving_dynamics_2/3(time) -> dv_driving_dynamics_2_time/1
  dbu_status_1/4(delta) -> dbu_status_1_delta/1
  res_initialization/2(status) -> res_initialization_status/1
  dv_driving_dynamics_2/1(signals) -> dv_driving_dynamics_2_bus/1
  dv_driving_dynamics_2/4(delta) -> dv_driving_dynamics_2_delta/1
  lv_bms_data_a/2(status) -> lv_bms_data_a_status/1
  dv_driving_dynamics_1/2(status) -> dv_driving_dynamics_1_status/1
  ams_status_1/4(delta) -> ams_status_1_delta/1
  dv_driving_dynamics_1/4(delta) -> dv_driving_dynamics_1_delta/1
  lv_bms_data_a/1(signals) -> lv_bms_data_a_bus/1
  set_mcu_inverter_points/3(time) -> set_mcu_inverter_points_time/1
  set_mcu_inverter_points/1(signals) -> set_mcu_inverter_points_bus/1
  set_mcu_inverter_points/4(delta) -> set_mcu_inverter_points_delta/1
  set_mcu_inverter_points/2(status) -> set_mcu_inverter_points_status/1

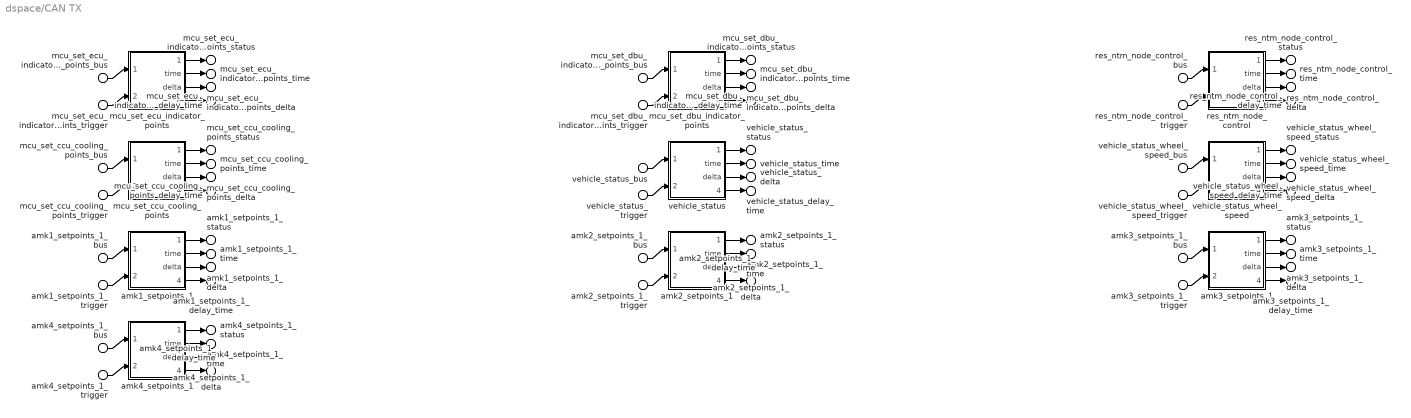
== system dspace/CAN TX ==
  mcu_set_ecu_indicator_points_bus : Inport  PortName=signals  Element=mcu_set_ecu_indicator_points
  mcu_set_dbu_indicator_points_bus : Inport  PortName=signals  Element=mcu_set_dbu_indicator_points
  res_ntm_node_control_bus : Inport  PortName=signals  Element=res_ntm_node_control
  mcu_set_ccu_cooling_points_bus : Inport  PortName=signals  Element=mcu_set_ccu_cooling_points
  vehicle_status_bus : Inport  PortName=signals  Element=vehicle_status
  vehicle_status_wheel_speed_bus : Inport  PortName=signals  Element=vehicle_status_wheel_speed
  amk1_setpoints_1_bus : Inport  PortName=signals  Element=amk1_setpoints_1
  amk2_setpoints_1_bus : Inport  PortName=signals  Element=amk2_setpoints_1
  amk3_setpoints_1_bus : Inport  PortName=signals  Element=amk3_setpoints_1
  amk4_setpoints_1_bus : Inport  PortName=signals  Element=amk4_setpoints_1
  mcu_set_ecu_indicator_points_trigger : Inport  Port=2  PortName=triggers  Element=mcu_set_ecu_indicator_points
  mcu_set_dbu_indicator_points_trigger : Inport  Port=2  PortName=triggers  Element=mcu_set_dbu_indicator_points
  res_ntm_node_control_trigger : Inport  Port=2  PortName=triggers  Element=res_ntm_node_control
  mcu_set_ccu_cooling_points_trigger : Inport  Port=2  PortName=triggers  Element=mcu_set_ccu_cooling_points
  vehicle_status_trigger : Inport  Port=2  PortName=triggers  Element=vehicle_status
  vehicle_status_wheel_speed_trigger : Inport  Port=2  PortName=triggers  Element=vehicle_status_wheel_speed
  amk1_setpoints_1_trigger : Inport  Port=2  PortName=triggers  Element=amk1_setpoints_1
  amk2_setpoints_1_trigger : Inport  Port=2  PortName=triggers  Element=amk2_setpoints_1
  amk3_setpoints_1_trigger : Inport  Port=2  PortName=triggers  Element=amk3_setpoints_1
  amk4_setpoints_1_trigger : Inport  Port=2  PortName=triggers  Element=amk4_setpoints_1
  amk1_setpoints_1 : Subsystem
  amk2_setpoints_1 : Subsystem
  amk3_setpoints_1 : Subsystem
  amk4_setpoints_1 : Subsystem
  mcu_set_ccu_cooling_points : Subsystem
  mcu_set_dbu_indicator_points : Subsystem
  mcu_set_ecu_indicator_points : Subsystem
  res_ntm_node_control : Subsystem
  vehicle_status : Subsystem
  vehicle_status_wheel_speed : Subsystem
  mcu_set_ecu_indicator_points_status : Outport  PortName=status  Element=mcu_set_ecu_indicator_points_status
  mcu_set_dbu_indicator_points_status : Outport  PortName=status  Element=mcu_set_dbu_indicator_points_status
  res_ntm_node_control_status : Outport  PortName=status  Element=res_ntm_node_control_status
  mcu_set_ccu_cooling_points_status : Outport  PortName=status  Element=mcu_set_ccu_cooling_points_status
  vehicle_status_status : Outport  PortName=status  Element=vehicle_status_status
  vehicle_status_wheel_speed_status : Outport  PortName=status  Element=vehicle_status_wheel_speed_status
  amk1_setpoints_1_status : Outport  PortName=status  Element=amk1_setpoints_1_status
  amk2_setpoints_1_status : Outport  PortName=status  Element=amk2_setpoints_1_status
  amk3_setpoints_1_status : Outport  PortName=status  Element=amk3_setpoints_1_status
  amk4_setpoints_1_status : Outport  PortName=status  Element=amk4_setpoints_1_status
  mcu_set_ecu_indicator_points_time : Outport  Port=2  PortName=time  Element=mcu_set_ecu_indicator_points_time
  mcu_set_dbu_indicator_points_time : Outport  Port=2  PortName=time  Element=mcu_set_dbu_indicator_points_time
  res_ntm_node_control_time : Outport  Port=2  PortName=time  Element=res_ntm_node_control_time
  mcu_set_ccu_cooling_points_time : Outport  Port=2  PortName=time  Element=mcu_set_ccu_cooling_points_time
  vehicle_status_time : Outport  Port=2  PortName=time  Element=vehicle_status_time
  vehicle_status_wheel_speed_time : Outport  Port=2  PortName=time  Element=vehicle_status_wheel_speed_time
  amk1_setpoints_1_time : Outport  Port=2  PortName=time  Element=amk1_setpoints_1_time
  amk2_setpoints_1_time : Outport  Port=2  PortName=time  Element=amk2_setpoints_1_time
  amk3_setpoints_1_time : Outport  Port=2  PortName=time  Element=amk3_setpoints_1_time
  amk4_setpoints_1_time : Outport  Port=2  PortName=time  Element=amk4_setpoints_1_time
  mcu_set_ecu_indicator_points_delta : Outport  Port=3  PortName=deltas  Element=mcu_set_ecu_indicator_points_delta
  mcu_set_dbu_indicator_points_delta : Outport  Port=3  PortName=deltas  Element=mcu_set_dbu_indicator_points_delta
  res_ntm_node_control_delta : Outport  Port=3  PortName=deltas  Element=res_ntm_node_control_delta
  mcu_set_ccu_cooling_points_delta : Outport  Port=3  PortName=deltas  Element=mcu_set_ccu_cooling_points_delta
  vehicle_status_delta : Outport  Port=3  PortName=deltas  Element=vehicle_status_delta
  vehicle_status_wheel_speed_delta : Outport  Port=3  PortName=deltas  Element=vehicle_status_wheel_speed_delta
  amk1_setpoints_1_delta : Outport  Port=3  PortName=deltas  Element=amk1_setpoints_1_delta
  amk2_setpoints_1_delta : Outport  Port=3  PortName=deltas  Element=amk2_setpoints_1_delta
  amk3_setpoints_1_delta : Outport  Port=3  PortName=deltas  Element=amk3_setpoints_1_delta
  amk4_setpoints_1_delta : Outport  Port=3  PortName=deltas  Element=amk4_setpoints_1_delta
  mcu_set_ecu_indicator_points_delay_time : Outport  Port=4  PortName=delay_time  Element=mcu_set_ecu_indicator_points_delay_time
  mcu_set_dbu_indicator_points_delay_time : Outport  Port=4  PortName=delay_time  Element=mcu_set_dbu_indicator_points_delay_time
  res_ntm_node_control_delay_time : Outport  Port=4  PortName=delay_time  Element=res_ntm_node_control_delay_time
  mcu_set_ccu_cooling_points_delay_time : Outport  Port=4  PortName=delay_time  Element=mcu_set_ccu_cooling_points_delay_time
  vehicle_status_delay_time : Outport  Port=4  PortName=delay_time  Element=vehicle_status_delay_time
  vehicle_status_wheel_speed_delay_time : Outport  Port=4  PortName=delay_time  Element=vehicle_status_wheel_speed_delay_time
  amk1_setpoints_1_delay_time : Outport  Port=4  PortName=delay_time  Element=amk1_setpoints_1_delay_time
  amk2_setpoints_1_delay_time : Outport  Port=4  PortName=delay_time  Element=amk2_setpoints_1_delay_time
  amk3_setpoints_1_delay_time : Outport  Port=4  PortName=delay_time  Element=amk3_setpoints_1_delay_time
  amk4_setpoints_1_delay_time : Outport  Port=4  PortName=delay_time  Element=amk4_setpoints_1_delay_time
  wires:
  mcu_set_ecu_indicator_points/1(status) -> mcu_set_ecu_indicator_points_status/1
  mcu_set_ecu_indicator_points/2(time) -> mcu_set_ecu_indicator_points_time/1
  mcu_set_ecu_indicator_points/3(delta) -> mcu_set_ecu_indicator_points_delta/1
  mcu_set_ecu_indicator_points/4(delay_time) -> mcu_set_ecu_indicator_points_delay_time/1
  mcu_set_ecu_indicator_points_bus/1 -> mcu_set_ecu_indicator_points/1(mcu_set_ecu_indicator_points)
  mcu_set_ecu_indicator_points_trigger/1 -> mcu_set_ecu_indicator_points/2(trigger)
  mcu_set_dbu_indicator_points/1(status) -> mcu_set_dbu_indicator_points_status/1
  mcu_set_dbu_indicator_points/2(time) -> mcu_set_dbu_indicator_points_time/1
  mcu_set_dbu_indicator_points/3(delta) -> mcu_set_dbu_indicator_points_delta/1
  mcu_set_dbu_indicator_points/4(delay_time) -> mcu_set_dbu_indicator_points_delay_time/1
  mcu_set_dbu_indicator_points_bus/1 -> mcu_set_dbu_indicator_points/1(mcu_set_dbu_indicator_points)
  mcu_set_dbu_indicator_points_trigger/1 -> mcu_set_dbu_indicator_points/2(trigger)
  res_ntm_node_control/1(status) -> res_ntm_node_control_status/1
  res_ntm_node_control/2(time) -> res_ntm_node_control_time/1
  res_ntm_node_control/3(delta) -> res_ntm_node_control_delta/1
  res_ntm_node_control/4(delay_time) -> res_ntm_node_control_delay_time/1
  res_ntm_node_control_bus/1 -> res_ntm_node_control/1(res_ntm_node_control)
  res_ntm_node_control_trigger/1 -> res_ntm_node_control/2(trigger)
  mcu_set_ccu_cooling_points/1(status) -> mcu_set_ccu_cooling_points_status/1
  mcu_set_ccu_cooling_points/2(time) -> mcu_set_ccu_cooling_points_time/1
  mcu_set_ccu_cooling_points/3(delta) -> mcu_set_ccu_cooling_points_delta/1
  mcu_set_ccu_cooling_points/4(delay_time) -> mcu_set_ccu_cooling_points_delay_time/1
  mcu_set_ccu_cooling_points_bus/1 -> mcu_set_ccu_cooling_points/1(mcu_set_ccu_cooling_points)
  mcu_set_ccu_cooling_points_trigger/1 -> mcu_set_ccu_cooling_points/2(trigger)
  vehicle_status/1(status) -> vehicle_status_status/1
  vehicle_status/2(time) -> vehicle_status_time/1
  vehicle_status/3(delta) -> vehicle_status_delta/1
  vehicle_status/4(delay_time) -> vehicle_status_delay_time/1
  vehicle_status_bus/1 -> vehicle_status/1(vehicle_status)
  vehicle_status_trigger/1 -> vehicle_status/2(trigger)
  vehicle_status_wheel_speed/1(status) -> vehicle_status_wheel_speed_status/1
  vehicle_status_wheel_speed/2(time) -> vehicle_status_wheel_speed_time/1
  vehicle_status_wheel_speed/3(delta) -> vehicle_status_wheel_speed_delta/1
  vehicle_status_wheel_speed/4(delay_time) -> vehicle_status_wheel_speed_delay_time/1
  vehicle_status_wheel_speed_bus/1 -> vehicle_status_wheel_speed/1(vehicle_status_wheel_speed)
  vehicle_status_wheel_speed_trigger/1 -> vehicle_status_wheel_speed/2(trigger)
  amk1_setpoints_1/1(status) -> amk1_setpoints_1_status/1
  amk1_setpoints_1/2(time) -> amk1_setpoints_1_time/1
  amk1_setpoints_1/3(delta) -> amk1_setpoints_1_delta/1
  amk1_setpoints_1/4(delay_time) -> amk1_setpoints_1_delay_time/1
  amk1_setpoints_1_bus/1 -> amk1_setpoints_1/1(amk1_setpoints_1)
  amk1_setpoints_1_trigger/1 -> amk1_setpoints_1/2(trigger)
  amk2_setpoints_1/1(status) -> amk2_setpoints_1_status/1
  amk2_setpoints_1/2(time) -> amk2_setpoints_1_time/1
  amk2_setpoints_1/3(delta) -> amk2_setpoints_1_delta/1
  amk2_setpoints_1/4(delay_time) -> amk2_setpoints_1_delay_time/1
  amk2_setpoints_1_bus/1 -> amk2_setpoints_1/1(amk2_setpoints_1)
  amk2_setpoints_1_trigger/1 -> amk2_setpoints_1/2(trigger)
  amk3_setpoints_1/1(status) -> amk3_setpoints_1_status/1
  amk3_setpoints_1/2(time) -> amk3_setpoints_1_time/1
  amk3_setpoints_1/3(delta) -> amk3_setpoints_1_delta/1
  amk3_setpoints_1/4(delay_time) -> amk3_setpoints_1_delay_time/1
  amk3_setpoints_1_bus/1 -> amk3_setpoints_1/1(amk3_setpoints_1)
  amk3_setpoints_1_trigger/1 -> amk3_setpoints_1/2(trigger)
  amk4_setpoints_1/1(status) -> amk4_setpoints_1_status/1
  amk4_setpoints_1/2(time) -> amk4_setpoints_1_time/1
  amk4_setpoints_1/3(delta) -> amk4_setpoints_1_delta/1
  amk4_setpoints_1/4(delay_time) -> amk4_setpoints_1_delay_time/1
  amk4_setpoints_1_bus/1 -> amk4_setpoints_1/1(amk4_setpoints_1)
  amk4_setpoints_1_trigger/1 -> amk4_setpoints_1/2(trigger)
